simulink model "Suspension_System"  (R2020b)
settings: Solver=VariableStepAuto  StartTime=0.0  StopTime=100  RelTol=1e-3
values from neighbouring files (symbols this model uses):
  b = 7    [data.m]
  k1 = 0.5    [data.m]
  k2 = 0.6    [data.m]
  m1 = 200    [data.m]
  m2 = 5    [data.m]
settings Model: Creator=vijay jagtap  LastModifiedBy=vijay jagtap

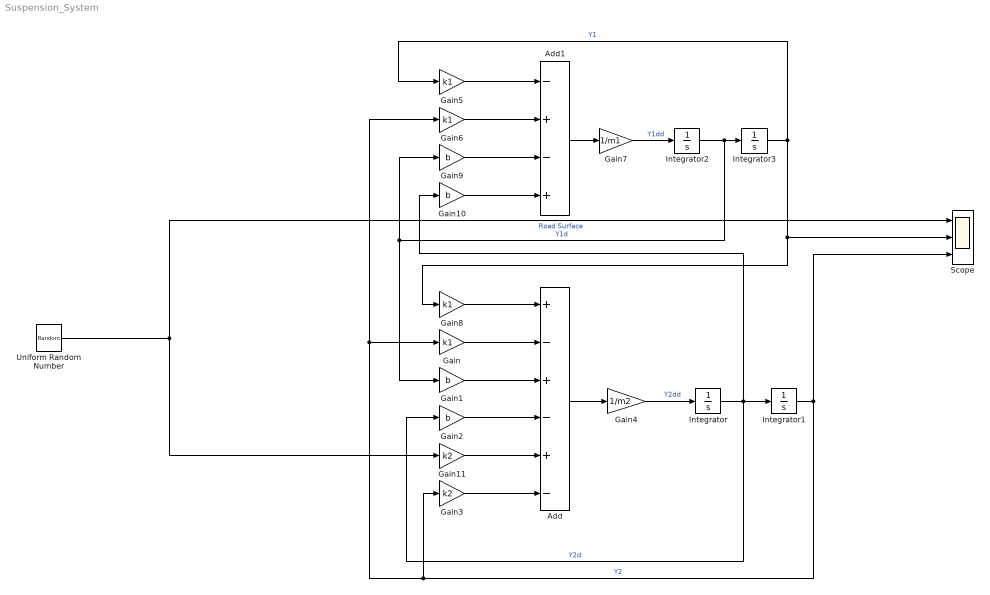
== system Suspension_System ==
  Add : Sum  Inputs=+-+-+-
  Add1 : Sum  Inputs=-+-+
  Gain{,5..6,8} (4 alike) : Gain  Gain=k1
  Gain{1..2,9..10} (4 alike) : Gain  Gain=b
  Gain11 : Gain  Gain=k2
  Gain3 : Gain  Gain=k2
  Gain4 : Gain  Gain=1/m2
  Gain7 : Gain  Gain=1/m1
  Integrator{,1..3} (4 alike) : Integrator
  Scope : Scope  NumInputPorts=3
  Uniform Random Number : UniformRandomNumber  SampleTime=0.1
  wires:
  Gain8/1 -> Add/1
  Gain3/1 -> Add/6
  Gain2/1 -> Add/4
  Gain1/1 -> Add/3
  Gain/1 -> Add/2
  Add/1 -> Gain4/1
  Gain4/1 -> Integrator/1  "Y2dd"
  Integrator/1 -> Gain10/1, Gain2/1, Integrator1/1  "Y2d"
  Gain6/1 -> Add1/2
  Gain5/1 -> Add1/1
  Add1/1 -> Gain7/1
  Gain7/1 -> Integrator2/1  "Y1dd"
  Integrator2/1 -> Gain1/1, Gain9/1, Integrator3/1  "Y1d"
  Integrator3/1 -> Gain8/1, Scope/2, Gain5/1  "Y1"
  Integrator1/1 -> Scope/3, Gain3/1, Gain6/1, Gain/1  "Y2"
  Gain9/1 -> Add1/3
  Gain10/1 -> Add1/4
  Uniform Random Number/1 -> Scope/1, Gain11/1  "Road Surface"
  Gain11/1 -> Add/5
